simulink model "ThrotModel_FirstPrincChamb_DataDrivenServoValve"  (R2025b)
settings: Solver=ode15s  StartTime=0.0  StopTime=10.0  RelTol=1e-3
values from neighbouring files (symbols this model uses):
  cstar_matr = readmatrix('cstar_lookup_table.xlsx','Range','C3:I23')    [cstar_lookup_table.m]
  OF_vec = readmatrix('cstar_lookup_table.xlsx','Range','C2:I2')    [cstar_lookup_table.m]    (also in sonvel_lookup_table.m = readmatrix('sonvel_lookup_table.xlsx','Range','C2:I2'))
  Pc_vec = psi_to_Pa*readmatrix('cstar_lookup_table.xlsx','Range','B3:B23')    [cstar_lookup_table.m]    (also in sonvel_lookup_table.m = psi_to_Pa*readmatrix('sonvel_lookup_table.xlsx','Range','B3:)
  psi_to_Pa = 6894.76    [cstar_lookup_table.m]    (also in sonvel_lookup_table.m)
  sonvel_matr = readmatrix('sonvel_lookup_table.xlsx','Range','C3:I23')    [sonvel_lookup_table.m]
undefined symbols (not defined in the file or in its folder): A_inj_f, A_inj_ox, A_t, Cd_inj_f_cstar_match, Cd_inj_ox_cstar_match, CdA_table, epsilon, k_servo, mdot_f_nom_cstar_match, OF, P_1_f, P_1_ox, P_amb, P_c_nom, P_c_ref_bp, rho_f, rho_ox, tau_servo, theta_bp, theta_ff_table, V_c
libraries: slpidlib x1
settings Model: Creator=gruby  LastModifiedBy=gruby

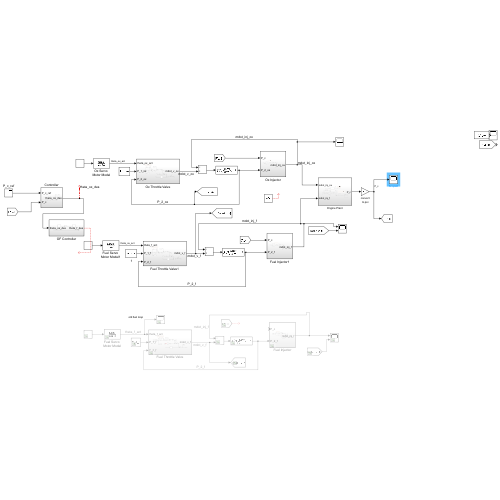
[thumbnail: Simulink's stored preview of the top-level diagram]
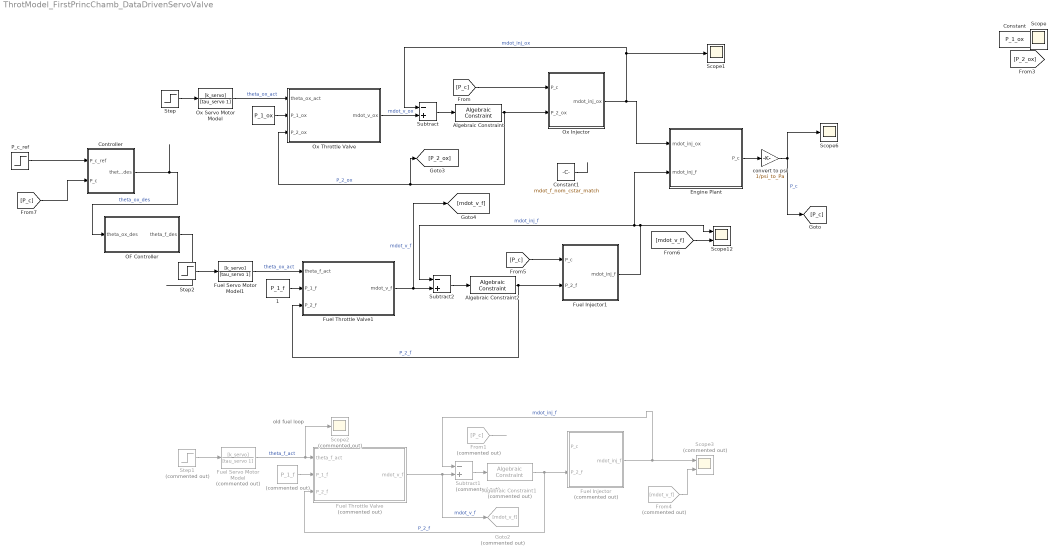
== system ThrotModel_FirstPrincChamb_DataDrivenServoValve ==
  note: old fuel loop
  " " : Constant  Value=P_1_ox
  "  " : Constant  Commented=on  Value=P_1_f
  " 1" : Constant  Value=P_1_f
  Algebraic Constraint : AlgebraicConstraint  InitialGuess=P_amb
  Algebraic Constraint1 : AlgebraicConstraint  Commented=on  InitialGuess=P_amb
  Algebraic Constraint2 : AlgebraicConstraint  InitialGuess=P_amb
  Constant : Constant  Value=P_1_ox
  Constant1 : Constant  Value=mdot_f_nom_cstar_match
  Controller : Subsystem
  Engine Plant : Subsystem
  From1 : From  Commented=on  GotoTag=P_c
  From4 : From  Commented=on  GotoTag=mdot_v_f
  Fuel Injector : Subsystem  Commented=on
  Fuel Injector1 : Subsystem
  Fuel Servo Motor Model : TransferFcn  Commented=on  Numerator=[k_servo]  Denominator=[tau_servo 1]
  Fuel Servo Motor Model1 : TransferFcn  Numerator=[k_servo]  Denominator=[tau_servo 1]
  Fuel Throttle Valve : Subsystem  Commented=on
  Fuel Throttle Valve1 : Subsystem
  Goto2 : Goto  Commented=on  GotoTag=mdot_v_f
  OF Controller : Subsystem
  Ox Injector : Subsystem
  Ox Servo Motor Model : TransferFcn  Numerator=[k_servo]  Denominator=[tau_servo 1]
  Ox Throttle Valve : Subsystem
  P_c_ref : Step  Before=P_amb  After=P_c_nom  SampleTime=0
  Scope : Scope
      settings: ActiveDisplayYMinimum=-194.92891097079226  ActiveDisplayYMaximum=779.85361280721634
  Scope1 : Scope
      settings: ActiveDisplayYMinimum=-0.017437742622917453  ActiveDisplayYMaximum=0.1569396836062571  DataLoggingVariableName=ScopeData13
  Scope12 : Scope  NumInputPorts=2
      settings: ActiveDisplayYMinimum=0.040994473538142895  ActiveDisplayYMaximum=0.067180844953612692  DataLoggingVariableName=ScopeData32
  Scope2 : Scope  Commented=on
      settings: ActiveDisplayYMinimum=-1  ActiveDisplayYMaximum=1  DataLoggingVariableName=ScopeData14
  Scope3 : Scope  Commented=on  NumInputPorts=2
      settings: ActiveDisplayYMinimum=0.047408074179886663  ActiveDisplayYMaximum=0.065021281191250752  DataLoggingVariableName=ScopeData3
  Scope6 : Scope
      settings: ActiveDisplayYMinimum=-5529.687087281246  ActiveDisplayYMaximum=974.03222862201051  YLabel=psi  DataLoggingVariableName=ScopeData25
  Step : Step  Time=5  Before=40  After=40  SampleTime=0
  Step1 : Step  Commented=on  Time=10  Before=50  After=50  SampleTime=0
  Step2 : Step  Time=5  Before=35  After=35  SampleTime=0
  Subtract : Sum  Inputs=-+
  Subtract1 : Sum  Commented=on  Inputs=-+
  Subtract2 : Sum  Inputs=-+
  convert to psi : Gain  Gain=1/psi_to_Pa
  wires:
  Ox Throttle Valve/1(mdot_v_ox) -> Subtract/2  "mdot_v_ox"
  Ox Injector/1(mdot_inj_ox) -> Engine Plant/1(mdot_inj_ox), Scope1/1, Subtract/1  "mdot_inj_ox"
  Fuel Injector/1(mdot_inj_f) -> Subtract1/1, Scope3/1  "mdot_inj_f"
  From1/1 -> ?
  Algebraic Constraint1/1 -> Fuel Injector/2(P_2_f), Fuel Throttle Valve/3(P_2_f)  "P_2_f"
  " "/1 -> Ox Throttle Valve/2(P_1_ox)
  "  "/1 -> Fuel Throttle Valve/2(P_1_f)
  Fuel Servo Motor Model/1 -> Scope2/1, Fuel Throttle Valve/1(theta_f_act)  "theta_f_act"
  Controller/1(theta_ox_des) -> OF Controller/1(theta_ox_des)  "theta_ox_des"
  P_c_ref/1 -> Controller/1(P_c_ref)
  Fuel Throttle Valve/1(mdot_v_f) -> Goto2/1, Subtract1/2  "mdot_v_f"
  Ox Servo Motor Model/1 -> Ox Throttle Valve/1(theta_ox_act)  "theta_ox_act"
  Subtract/1 -> Algebraic Constraint/1
  Algebraic Constraint/1 -> [P_2_ox], Ox Throttle Valve/3(P_2_ox), Ox Injector/2(P_2_ox)  "P_2_ox"
  Subtract1/1 -> Algebraic Constraint1/1
  Engine Plant/1(P_c) -> convert to psi/1
  convert to psi/1 -> [P_c], Scope6/1  "P_c"
  [P_c] -> Ox Injector/1(P_c)
  Step1/1 -> Fuel Servo Motor Model/1
  From4/1 -> Scope3/2
  " 1"/1 -> Fuel Throttle Valve1/2(P_1_f)
  OF Controller/1(theta_f_des) -> ?
  Fuel Throttle Valve1/1(mdot_v_f) -> [mdot_v_f], Subtract2/2  "mdot_v_f"
  Subtract2/1 -> Algebraic Constraint2/1
  Algebraic Constraint2/1 -> Fuel Throttle Valve1/3(P_2_f), Fuel Injector1/2(P_2_f)  "P_2_f"
  Fuel Injector1/1(mdot_inj_f) -> Engine Plant/2(mdot_inj_f), Subtract2/1, Scope12/1  "mdot_inj_f"
  Fuel Servo Motor Model1/1 -> Fuel Throttle Valve1/1(theta_f_act)  "theta_ox_act"
  [P_c] -> Fuel Injector1/1(P_c)
  [mdot_v_f] -> Scope12/2
  [P_c] -> Controller/2(P_c)
  Step/1 -> Ox Servo Motor Model/1
  Constant1/1 -> ?
  Step2/1 -> Fuel Servo Motor Model1/1

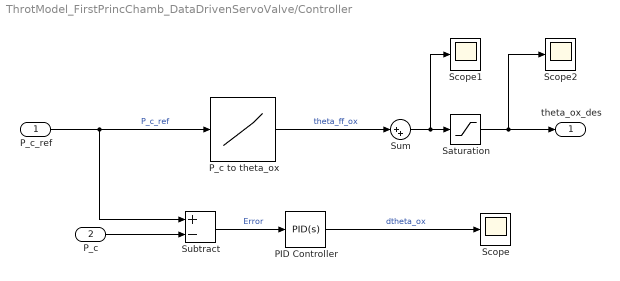
== system ThrotModel_FirstPrincChamb_DataDrivenServoValve/Controller ==
  P_c_ref : Inport
  P_c : Inport  Port=2
  PID Controller : slpidlib/PID Controller  Controller=PID  Form=Parallel  TimeDomain=Continuous-time  UseExternalTs=off  SampleTime=-1  IntegratorMethod=Forward Euler  FilterMethod=Forward Euler  ControllerParametersSource=internal  P=1  I=.1  UseKiTs=off  D=0  UseExternalDerivativeSource=off  N=100  UseFilter=on  TunerSelectOption=Transfer Function Based (PID Tuner App)  InitialConditionSource=internal  InitialConditionForIntegrator=0  InitialConditionForFilter=0  DifferentiatorICPrevScaledInput=0  ExternalReset=none  TrackingMode=off  Kt=1  LimitOutput=off  SatLimitsSource=internal  UpperSaturationLimit=inf  LowerSaturationLimit=-inf  LinearizeAsGain=on  AntiWindupMode=none  Kb=1  LimitIntegrator=off  UpperIntegratorSaturationLimit=inf  LowerIntegratorSaturationLimit=-inf  POutMin=[]  POutMax=[]  IOutMin=[]  IOutMax=[]  DOutMin=[]  DOutMax=[]  NOutMin=[]  NOutMax=[]  SumOutMin=[]  SumOutMax=[]  SaturationOutMin=[]  SaturationOutMax=[]  PParamMin=[]  PParamMax=[]  IParamMin=[]  IParamMax=[]  DParamMin=[]  DParamMax=[]  NParamMin=[]  NParamMax=[]  KbParamMin=[]  KbParamMax=[]  KtParamMin=[]  KtParamMax=[]  KbOutMin=[]  KbOutMax=[]  KtOutMin=[]  KtOutMax=[]  IntegratorOutMin=[]  IntegratorOutMax=[]  FilterOutMin=[]  FilterOutMax=[]  SumI1OutMin=[]  SumI1OutMax=[]  SumI2OutMin=[]  SumI2OutMax=[]  SumI3OutMin=[]  SumI3OutMax=[]  SumI4OutMin=[]  SumI4OutMax=[]  SumDOutMin=[]  SumDOutMax=[]  DifferentiatorOutMin=[]  DifferentiatorOutMax=[]  FilterDiffOutCoefMin=[]  FilterDiffOutCoefMax=[]  ReciprocalOutMin=[]  ReciprocalOutMax=[]  SumDenOutMin=[]  SumDenOutMax=[]  SumNumOutMin=[]  SumNumOutMax=[]  DivideOutMin=[]  DivideOutMax=[]  UdiffTsProdOutMin=[]  UdiffTsProdOutMax=[]  NTsProdOutMin=[]  NTsProdOutMax=[]  UintegralTsProdOutMin=[]  UintegralTsProdOutMax=[]  UngainTsProdOutMin=[]  UngainTsProdOutMax=[]  ClampingZeroOutDataTypeStr=Inherit: Inherit via back propagation  ClampingZeroOutMin=[]  ClampingZeroOutMax=[]  FilterDenConstantOutDataTypeStr=Inherit: Inherit via back propagation  FilterDenConstantOutMin=[]  FilterDenConstantOutMax=[]  PCopyOutDataTypeStr=Inherit: Inherit via back propagation  PCopyOutMin=[]  PCopyOutMax=[]  NCopyOutDataTypeStr=Inherit: Inherit via back propagation  NCopyOutMin=[]  NCopyOutMax=[]  IntegratorContinuousStateAttributes=''  IntegratorStateMustResolveToSignalObject=off  IntegratorRTWStateStorageClass=Auto  FilterContinuousStateAttributes=''  FilterStateMustResolveToSignalObject=off  FilterRTWStateStorageClass=Auto  ParallelPVariant=InternalParameters  IdealPVariant=Disabled  IVariant=InternalParameters  DVariant=InternalParameters  IntegratorVariant=Continuous  SatVariant=Disabled  AWVariant=Passthrough  PCopyVariant=Disabled  TRVariant=Disabled  FdbkBlocksVariant=Forward  IdealPFdbkVariant=Disabled  SatFdbkVariant=Disabled  DerivativeFilterVariant=ContFilter  NVariant=InternalParameters  NCopyVariant=Disabled  FilterICVariant=InternalICsFilter  IntegratorICVariant=InternalICs  ExternalResetVariant=Disabled  TRSumVariant=Passthrough  SumFdbkVariant=Disabled  SumVariant=Sum_PID  TsampFilterVariant=InternalTs  TsampNgainVariant=Passthrough  TsampIntegralVariant=Disabled_SignalSpec  ExternalSaturationOutDataTypeStr=Inherit: Same as second input  DerivativeSourceVariant=ErrorSignal  PreIntVariant=InternalPreInt
  P_c to theta_ox : Lookup_n-D  NumberOfTableDimensions=1  BreakpointsForDimension1=P_c_ref_bp  Table=theta_ff_table  ExtrapMethod=Clip  UseLastTableValue=on  InternalRulePriority=Speed  RndMeth=Simplest
  Saturation : Saturate  UpperLimit=60  LowerLimit=0
  Scope : Scope
      settings: ActiveDisplayYMinimum=-1  ActiveDisplayYMaximum=1  DataLoggingVariableName=ScopeData4
  Scope1 : Scope
      settings: ActiveDisplayYMinimum=-1  ActiveDisplayYMaximum=1  DataLoggingVariableName=ScopeData5
  Scope2 : Scope
      settings: ActiveDisplayYMinimum=-1  ActiveDisplayYMaximum=1  DataLoggingVariableName=ScopeData7
  Subtract : Sum  Inputs=+-
  Sum : Sum  Inputs=|++
  theta_ox_des : Outport
  wires:
  P_c_ref/1 -> Subtract/1, P_c to theta_ox/1  "P_c_ref"
  P_c to theta_ox/1 -> Sum/1  "theta_ff_ox"
  P_c/1 -> Subtract/2
  Subtract/1 -> PID Controller/1  "Error"
  PID Controller/1 -> Scope/1  "dtheta_ox"
  Sum/1 -> Saturation/1, Scope1/1
  Saturation/1 -> Scope2/1, theta_ox_des/1

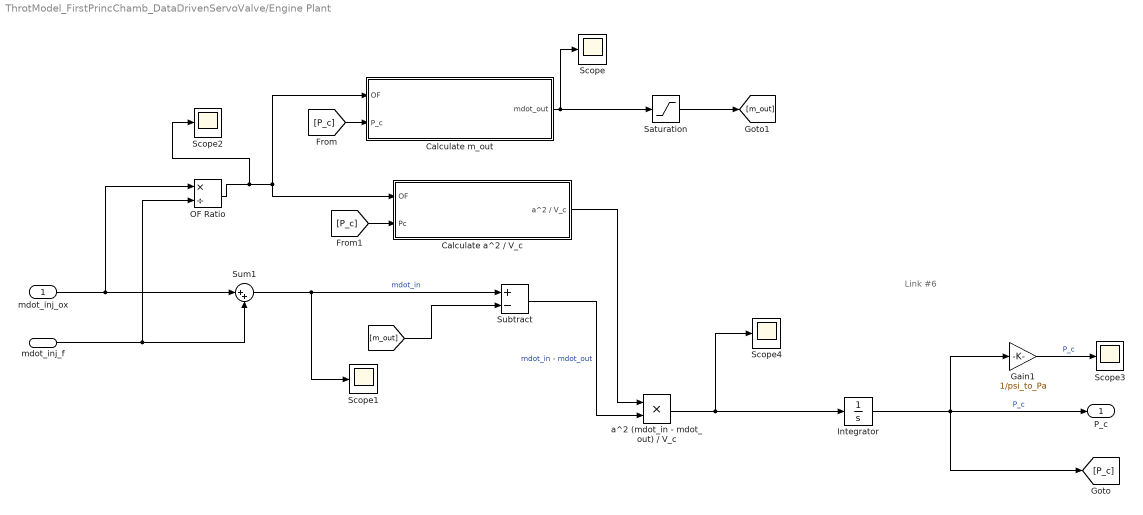
== system ThrotModel_FirstPrincChamb_DataDrivenServoValve/Engine Plant ==
  note: Link #6
  mdot_inj_ox : Inport
  mdot_inj_f : Inport  Port=2
  Calculate a^2 / V_c : Subsystem
  Calculate m_out : Subsystem
  Gain1 : Gain  Gain=1/psi_to_Pa
  Integrator : Integrator  InitialCondition=P_amb
  OF Ratio : Product  Inputs=*/
  Saturation : Saturate  UpperLimit=+Inf  LowerLimit=1e-8
  Scope{,1..4} (5 alike) : Scope
      Scope settings: ActiveDisplayYMinimum=-0.12055237902369925  ActiveDisplayYMaximum=0.74421105640453378  DataLoggingVariableName=ScopeData16
      Scope1 settings: ActiveDisplayYMinimum=0.43926765376755966  ActiveDisplayYMaximum=0.43944760494726304  DataLoggingVariableName=ScopeData17
      Scope2 settings: ActiveDisplayYMinimum=-1  ActiveDisplayYMaximum=1  DataLoggingVariableName=ScopeData15
      Scope3 settings: ActiveDisplayYMinimum=585.13756667691121  ActiveDisplayYMaximum=610.588561189296  DataLoggingVariableName=ScopeData28
      Scope4 settings: ActiveDisplayYMinimum=-1  ActiveDisplayYMaximum=1  DataLoggingVariableName=ScopeData29
  Subtract : Sum  Inputs=+-
  Sum1 : Sum  Inputs=|++
  "a^2 (mdot_in - mdot_out) / V_c " : Product
  P_c : Outport
  wires:
  mdot_inj_f/1 -> OF Ratio/2, Sum1/2
  mdot_inj_ox/1 -> OF Ratio/1, Sum1/1
  Integrator/1 -> Gain1/1, P_c/1, [P_c]  "P_c"
  OF Ratio/1 -> Scope2/1, Calculate a^2 / V_c/1(OF), Calculate m_out/1(OF)
  [P_c] -> Calculate m_out/2(P_c)
  [P_c] -> Calculate a^2 / V_c/2(Pc)
  Calculate a^2 / V_c/1(a^2 / V_c) -> "a^2 (mdot_in - mdot_out) / V_c "/1
  Calculate m_out/1(mdot_out) -> Scope/1, Saturation/1
  [m_out] -> Subtract/2
  Sum1/1 -> Scope1/1, Subtract/1  "mdot_in"
  Subtract/1 -> "a^2 (mdot_in - mdot_out) / V_c "/2  "mdot_in - mdot_out"
  Saturation/1 -> [m_out]
  "a^2 (mdot_in - mdot_out) / V_c "/1 -> Integrator/1, Scope4/1
  Gain1/1 -> Scope3/1  "P_c"

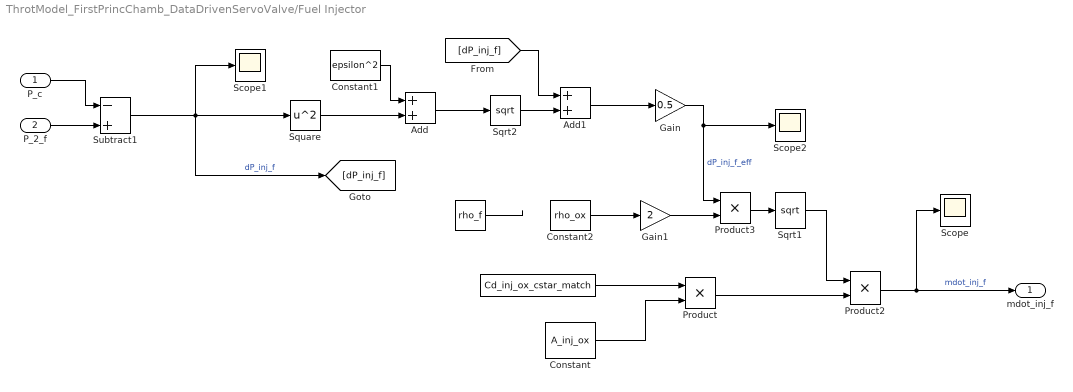
== system ThrotModel_FirstPrincChamb_DataDrivenServoValve/Fuel Injector ==
  P_c : Inport
  P_2_f : Inport  Port=2
  "  " : Constant  Value=Cd_inj_ox_cstar_match
  "    " : Constant  Value=rho_f
  Add : Sum
  Add1 : Sum
  Constant : Constant  Value=A_inj_ox
  Constant1 : Constant  Value=epsilon^2
  Constant2 : Constant  Value=rho_ox
  Gain : Gain  Gain=0.5
  Gain1 : Gain  Gain=2
  Product : Product
  Product2 : Product
  Product3 : Product
  Scope : Scope
      settings: ActiveDisplayYMinimum=-1  ActiveDisplayYMaximum=1  DataLoggingVariableName=ScopeData8
  Scope1 : Scope
      settings: DataLoggingVariableName=ScopeData9
  Scope2 : Scope
      settings: DataLoggingVariableName=ScopeData22
  Sqrt1 : Sqrt
  Sqrt2 : Sqrt
  Square : Math  Operator=square
  Subtract1 : Sum  Inputs=-+
  mdot_inj_f : Outport
  wires:
  Subtract1/1 -> [dP_inj_f], Square/1, Scope1/1  "dP_inj_f"
  "    "/1 -> ?
  P_2_f/1 -> Subtract1/2
  Product3/1 -> Sqrt1/1
  Sqrt1/1 -> Product2/1
  Gain1/1 -> Product3/2
  P_c/1 -> Subtract1/1
  Product2/1 -> Scope/1, mdot_inj_f/1  "mdot_inj_f"
  "  "/1 -> Product/1
  Product/1 -> Product2/2
  Constant/1 -> Product/2
  Constant1/1 -> Add/1
  [dP_inj_f] -> Add1/1
  Sqrt2/1 -> Add1/2
  Add/1 -> Sqrt2/1
  Square/1 -> Add/2
  Add1/1 -> Gain/1
  Gain/1 -> Product3/1, Scope2/1  "dP_inj_f_eff"
  Constant2/1 -> Gain1/1

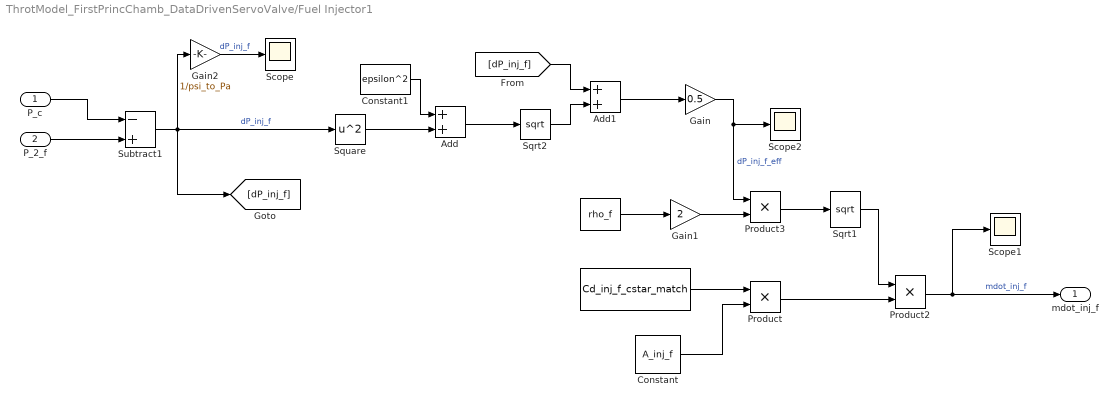
== system ThrotModel_FirstPrincChamb_DataDrivenServoValve/Fuel Injector1 ==
  P_c : Inport
  P_2_f : Inport  Port=2
  " " : Constant  Value=rho_f
  "    " : Constant  Value=Cd_inj_f_cstar_match
  Add : Sum
  Add1 : Sum
  Constant : Constant  Value=A_inj_f
  Constant1 : Constant  Value=epsilon^2
  Gain : Gain  Gain=0.5
  Gain1 : Gain  Gain=2
  Gain2 : Gain  Gain=1/psi_to_Pa
  Product : Product
  Product2 : Product
  Product3 : Product
  Scope : Scope
      settings: ActiveDisplayYMinimum=349.39624519430527  ActiveDisplayYMaximum=354.86657235471296
  Scope1 : Scope
      settings: ActiveDisplayYMinimum=-1  ActiveDisplayYMaximum=1  DataLoggingVariableName=ScopeData2
  Scope2 : Scope
      settings: DataLoggingVariableName=ScopeData21
  Sqrt1 : Sqrt
  Sqrt2 : Sqrt
  Square : Math  Operator=square
  Subtract1 : Sum  Inputs=-+
  mdot_inj_f : Outport
  wires:
  Subtract1/1 -> Gain2/1, [dP_inj_f], Square/1  "dP_inj_f"
  "    "/1 -> Product/1
  " "/1 -> Gain1/1
  P_2_f/1 -> Subtract1/2
  Product3/1 -> Sqrt1/1
  Sqrt1/1 -> Product2/1
  Gain1/1 -> Product3/2
  P_c/1 -> Subtract1/1
  Product2/1 -> Scope1/1, mdot_inj_f/1  "mdot_inj_f"
  Constant/1 -> Product/2
  Product/1 -> Product2/2
  Add1/1 -> Gain/1
  Sqrt2/1 -> Add1/2
  Add/1 -> Sqrt2/1
  [dP_inj_f] -> Add1/1
  Constant1/1 -> Add/1
  Square/1 -> Add/2
  Gain/1 -> Product3/1, Scope2/1  "dP_inj_f_eff"
  Gain2/1 -> Scope/1  "dP_inj_f"

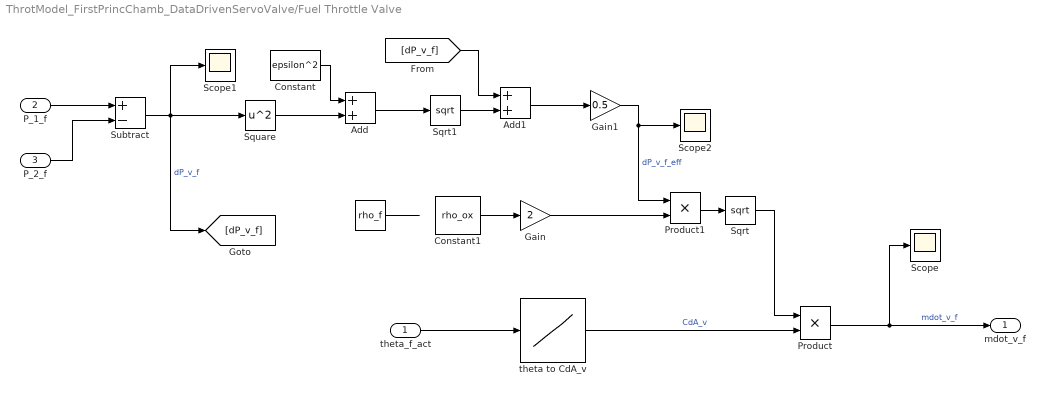
== system ThrotModel_FirstPrincChamb_DataDrivenServoValve/Fuel Throttle Valve ==
  theta_f_act : Inport
  P_1_f : Inport  Port=2
  P_2_f : Inport  Port=3
  "  " : Constant  Value=rho_f
  Add : Sum
  Add1 : Sum
  Constant : Constant  Value=epsilon^2
  Constant1 : Constant  Value=rho_ox
  Gain : Gain  Gain=2
  Gain1 : Gain  Gain=0.5
  Product : Product
  Product1 : Product
  Scope : Scope
      settings: DataLoggingVariableName=ScopeData11
  Scope1 : Scope
      settings: ActiveDisplayYMinimum=-1  ActiveDisplayYMaximum=1  DataLoggingVariableName=ScopeData12
  Scope2 : Scope
      settings: DataLoggingVariableName=ScopeData20
  Sqrt : Sqrt
  Sqrt1 : Sqrt
  Square : Math  Operator=square
  Subtract : Sum  Inputs=+-
  theta to CdA_v : Lookup_n-D  NumberOfTableDimensions=1  BreakpointsForDimension1=theta_bp  Table=CdA_table  ExtrapMethod=Clip  UseLastTableValue=on  InternalRulePriority=Speed  RndMeth=Simplest
  mdot_v_f : Outport
  wires:
  Sqrt/1 -> Product/1
  "  "/1 -> ?
  Product/1 -> Scope/1, mdot_v_f/1  "mdot_v_f"
  Gain/1 -> Product1/2
  theta to CdA_v/1 -> Product/2  "CdA_v"
  Product1/1 -> Sqrt/1
  theta_f_act/1 -> theta to CdA_v/1
  P_2_f/1 -> Subtract/2
  P_1_f/1 -> Subtract/1
  Sqrt1/1 -> Add1/2
  Add/1 -> Sqrt1/1
  [dP_v_f] -> Add1/1
  Constant/1 -> Add/1
  Subtract/1 -> [dP_v_f], Square/1, Scope1/1  "dP_v_f"
  Square/1 -> Add/2
  Add1/1 -> Gain1/1
  Gain1/1 -> Product1/1, Scope2/1  "dP_v_f_eff"
  Constant1/1 -> Gain/1

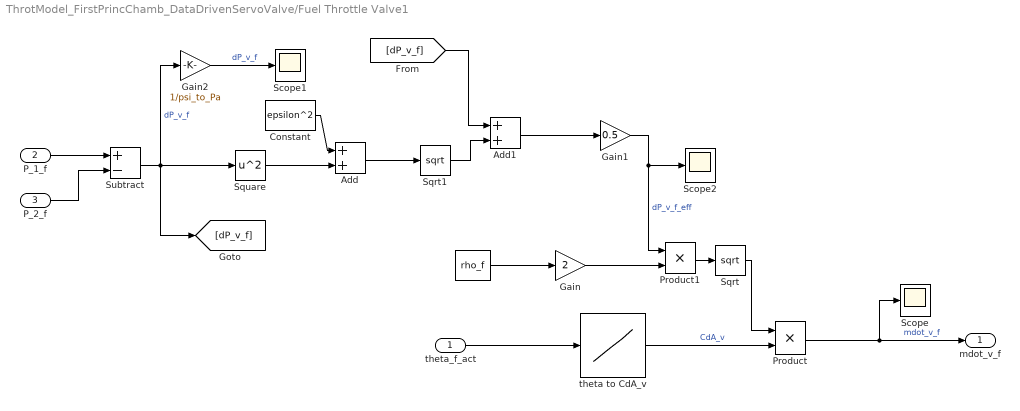
== system ThrotModel_FirstPrincChamb_DataDrivenServoValve/Fuel Throttle Valve1 ==
  theta_f_act : Inport
  P_1_f : Inport  Port=2
  P_2_f : Inport  Port=3
  "  " : Constant  Value=rho_f
  Add : Sum
  Add1 : Sum
  Constant : Constant  Value=epsilon^2
  Gain : Gain  Gain=2
  Gain1 : Gain  Gain=0.5
  Gain2 : Gain  Gain=1/psi_to_Pa
  Product : Product
  Product1 : Product
  Scope : Scope
      settings: ActiveDisplayYMinimum=-1  ActiveDisplayYMaximum=1  DataLoggingVariableName=ScopeData6
  Scope1 : Scope
      settings: ActiveDisplayYMinimum=67.114933050703414  ActiveDisplayYMaximum=247.40272483791119  DataLoggingVariableName=ScopeData10
  Scope2 : Scope
      settings: ActiveDisplayYMinimum=-1  ActiveDisplayYMaximum=1  DataLoggingVariableName=ScopeData19
  Sqrt : Sqrt
  Sqrt1 : Sqrt
  Square : Math  Operator=square
  Subtract : Sum  Inputs=+-
  theta to CdA_v : Lookup_n-D  NumberOfTableDimensions=1  BreakpointsForDimension1=theta_bp  Table=CdA_table  ExtrapMethod=Clip  UseLastTableValue=on  InternalRulePriority=Speed  RndMeth=Simplest
  mdot_v_f : Outport
  wires:
  Subtract/1 -> Gain2/1, [dP_v_f], Square/1  "dP_v_f"
  Sqrt/1 -> Product/1
  "  "/1 -> Gain/1
  Product/1 -> Scope/1, mdot_v_f/1  "mdot_v_f"
  Gain/1 -> Product1/2
  theta to CdA_v/1 -> Product/2  "CdA_v"
  Product1/1 -> Sqrt/1
  theta_f_act/1 -> theta to CdA_v/1
  P_1_f/1 -> Subtract/1
  P_2_f/1 -> Subtract/2
  Square/1 -> Add/2
  Constant/1 -> Add/1
  Add/1 -> Sqrt1/1
  [dP_v_f] -> Add1/1
  Sqrt1/1 -> Add1/2
  Add1/1 -> Gain1/1
  Gain1/1 -> Product1/1, Scope2/1  "dP_v_f_eff"
  Gain2/1 -> Scope1/1  "dP_v_f"

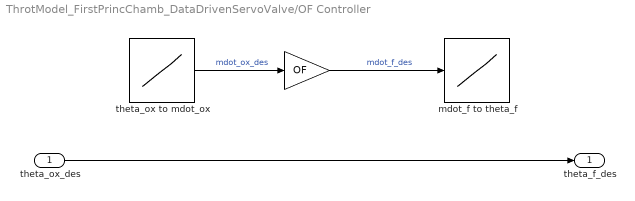
== system ThrotModel_FirstPrincChamb_DataDrivenServoValve/OF Controller ==
  theta_ox_des : Inport
  " " : Gain  Gain=OF
  mdot_f to theta_f : Lookup_n-D  NumberOfTableDimensions=1  BreakpointsForDimension1=[-5:5]  Table=tanh([-5:5])  InternalRulePriority=Speed  RndMeth=Simplest
  theta_ox to mdot_ox : Lookup_n-D  NumberOfTableDimensions=1  BreakpointsForDimension1=[-5:5]  Table=tanh([-5:5])  InternalRulePriority=Speed  RndMeth=Simplest
  theta_f_des : Outport
  wires:
  theta_ox_des/1 -> theta_f_des/1
  theta_ox to mdot_ox/1 -> " "/1  "mdot_ox_des"
  " "/1 -> mdot_f to theta_f/1  "mdot_f_des"

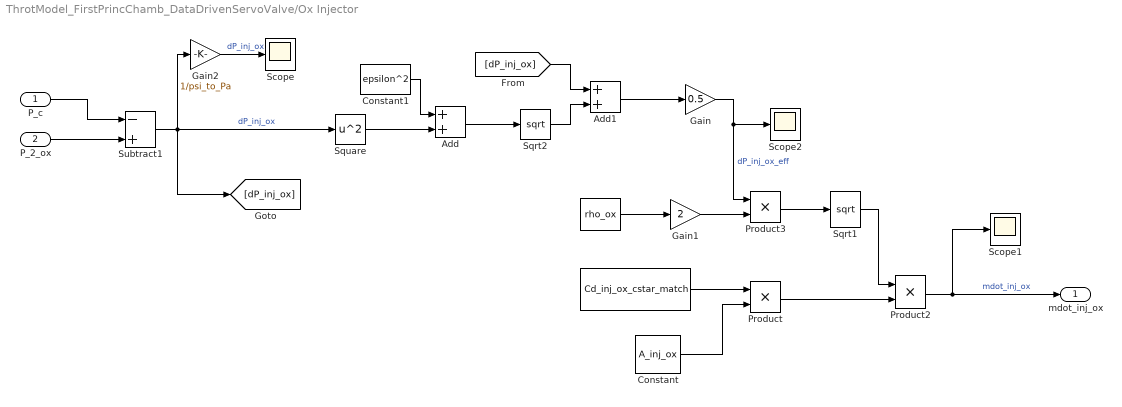
== system ThrotModel_FirstPrincChamb_DataDrivenServoValve/Ox Injector ==
  P_c : Inport
  P_2_ox : Inport  Port=2
  " " : Constant  Value=rho_ox
  "    " : Constant  Value=Cd_inj_ox_cstar_match
  Add : Sum
  Add1 : Sum
  Constant : Constant  Value=A_inj_ox
  Constant1 : Constant  Value=epsilon^2
  Gain : Gain  Gain=0.5
  Gain1 : Gain  Gain=2
  Gain2 : Gain  Gain=1/psi_to_Pa
  Product : Product
  Product2 : Product
  Product3 : Product
  Scope : Scope
      settings: ActiveDisplayYMinimum=349.39624519430527  ActiveDisplayYMaximum=354.86657235471296
  Scope1 : Scope
      settings: ActiveDisplayYMinimum=-1  ActiveDisplayYMaximum=1  DataLoggingVariableName=ScopeData2
  Scope2 : Scope
      settings: DataLoggingVariableName=ScopeData21
  Sqrt1 : Sqrt
  Sqrt2 : Sqrt
  Square : Math  Operator=square
  Subtract1 : Sum  Inputs=-+
  mdot_inj_ox : Outport
  wires:
  Subtract1/1 -> Gain2/1, [dP_inj_ox], Square/1  "dP_inj_ox"
  "    "/1 -> Product/1
  " "/1 -> Gain1/1
  P_2_ox/1 -> Subtract1/2
  Product3/1 -> Sqrt1/1
  Sqrt1/1 -> Product2/1
  Gain1/1 -> Product3/2
  P_c/1 -> Subtract1/1
  Product2/1 -> Scope1/1, mdot_inj_ox/1  "mdot_inj_ox"
  Constant/1 -> Product/2
  Product/1 -> Product2/2
  Add1/1 -> Gain/1
  Sqrt2/1 -> Add1/2
  Add/1 -> Sqrt2/1
  [dP_inj_ox] -> Add1/1
  Constant1/1 -> Add/1
  Square/1 -> Add/2
  Gain/1 -> Product3/1, Scope2/1  "dP_inj_ox_eff"
  Gain2/1 -> Scope/1  "dP_inj_ox"

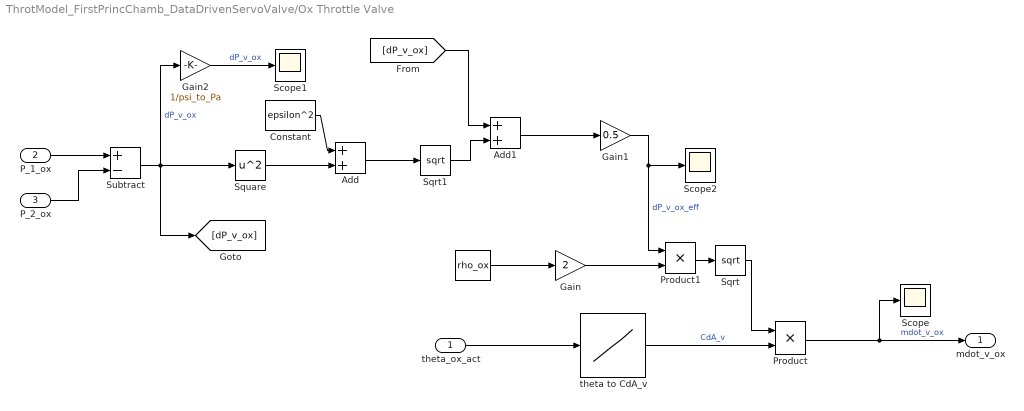
== system ThrotModel_FirstPrincChamb_DataDrivenServoValve/Ox Throttle Valve ==
  theta_ox_act : Inport
  P_1_ox : Inport  Port=2
  P_2_ox : Inport  Port=3
  "  " : Constant  Value=rho_ox
  Add : Sum
  Add1 : Sum
  Constant : Constant  Value=epsilon^2
  Gain : Gain  Gain=2
  Gain1 : Gain  Gain=0.5
  Gain2 : Gain  Gain=1/psi_to_Pa
  Product : Product
  Product1 : Product
  Scope : Scope
      settings: ActiveDisplayYMinimum=-1  ActiveDisplayYMaximum=1  DataLoggingVariableName=ScopeData6
  Scope1 : Scope
      settings: ActiveDisplayYMinimum=67.114933050703414  ActiveDisplayYMaximum=247.40272483791119  DataLoggingVariableName=ScopeData10
  Scope2 : Scope
      settings: ActiveDisplayYMinimum=-1  ActiveDisplayYMaximum=1  DataLoggingVariableName=ScopeData19
  Sqrt : Sqrt
  Sqrt1 : Sqrt
  Square : Math  Operator=square
  Subtract : Sum  Inputs=+-
  theta to CdA_v : Lookup_n-D  NumberOfTableDimensions=1  BreakpointsForDimension1=theta_bp  Table=CdA_table  ExtrapMethod=Clip  UseLastTableValue=on  InternalRulePriority=Speed  RndMeth=Simplest
  mdot_v_ox : Outport
  wires:
  Subtract/1 -> Gain2/1, [dP_v_ox], Square/1  "dP_v_ox"
  Sqrt/1 -> Product/1
  "  "/1 -> Gain/1
  Product/1 -> Scope/1, mdot_v_ox/1  "mdot_v_ox"
  Gain/1 -> Product1/2
  theta to CdA_v/1 -> Product/2  "CdA_v"
  Product1/1 -> Sqrt/1
  theta_ox_act/1 -> theta to CdA_v/1
  P_1_ox/1 -> Subtract/1
  P_2_ox/1 -> Subtract/2
  Square/1 -> Add/2
  Constant/1 -> Add/1
  Add/1 -> Sqrt1/1
  [dP_v_ox] -> Add1/1
  Sqrt1/1 -> Add1/2
  Add1/1 -> Gain1/1
  Gain1/1 -> Product1/1, Scope2/1  "dP_v_ox_eff"
  Gain2/1 -> Scope1/1  "dP_v_ox"

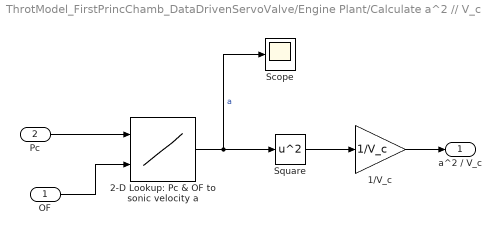
== system ThrotModel_FirstPrincChamb_DataDrivenServoValve/Engine Plant/Calculate a^2 // V_c ==
  OF : Inport
  Pc : Inport  Port=2
  1/V_c : Gain  Gain=1/V_c
  2-D Lookup: Pc & OF to sonic velocity a : Lookup_n-D  BreakpointsForDimension1=Pc_vec  BreakpointsForDimension2=OF_vec  Table=sonvel_matr  ExtrapMethod=Clip  UseLastTableValue=on  InternalRulePriority=Speed  RndMeth=Simplest
      settings: InputPortMap=u0,u1
  Scope : Scope
      settings: ActiveDisplayYMinimum=-1  ActiveDisplayYMaximum=1  DataLoggingVariableName=ScopeData15
  Square : Math  Operator=square
  a^2 / V_c : Outport
  wires:
  2-D Lookup: Pc & OF to sonic velocity a/1 -> Scope/1, Square/1  "a"
  Square/1 -> 1/V_c/1
  1/V_c/1 -> a^2 / V_c/1
  OF/1 -> 2-D Lookup: Pc & OF to sonic velocity a/2
  Pc/1 -> 2-D Lookup: Pc & OF to sonic velocity a/1

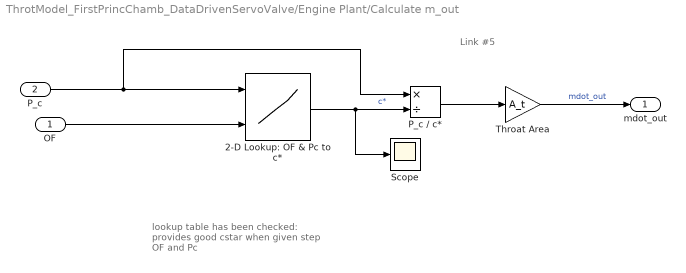
== system ThrotModel_FirstPrincChamb_DataDrivenServoValve/Engine Plant/Calculate m_out ==
  note: lookup table has been checked: provides good cstar when given step OF and Pc
  note: Link #5
  OF : Inport
  P_c : Inport  Port=2
  2-D Lookup: OF & Pc to c* : Lookup_n-D  BreakpointsForDimension1=Pc_vec  BreakpointsForDimension2=OF_vec  Table=cstar_matr  ExtrapMethod=Clip  UseLastTableValue=on  InternalRulePriority=Speed  RndMeth=Simplest
      settings: InputPortMap=u0,u1
  P_c / c* : Product  Inputs=*/
  Scope : Scope
      settings: ActiveDisplayYMinimum=-1  ActiveDisplayYMaximum=1  DataLoggingVariableName=ScopeData24
  Throat Area : Gain  Gain=A_t
  mdot_out : Outport
  wires:
  2-D Lookup: OF & Pc to c*/1 -> Scope/1, P_c / c*/2  "c*"
  P_c / c*/1 -> Throat Area/1
  OF/1 -> 2-D Lookup: OF & Pc to c*/2
  Throat Area/1 -> mdot_out/1  "mdot_out"
  P_c/1 -> P_c / c*/1, 2-D Lookup: OF & Pc to c*/1
